simulink model "Octacopter"  (R2022b)
settings: Solver=VariableStepAuto  StartTime=0.0  StopTime=sim_time  RelTol=1e-3
values from neighbouring files (symbols this model uses):
  b = 1.2953*1e-5    (= 1.2953e-05)    [Junesh_Octacopter.m]    (also in Junesh_Octacopter.mat)
  d = 0.008    [Junesh_Octacopter.m]    (also in Junesh_Octacopter.mat)
  g = 9.81    [Junesh_Octacopter.m]    (also in Junesh_Octacopter.mat)
  Ixx = 0.0820    (= 0.082)    [Junesh_Octacopter.m]    (also in Junesh_Octacopter.mat)
  Iyy = 0.0845    [Junesh_Octacopter.m]    (also in Junesh_Octacopter.mat)
  Izz = 0.1377    [Junesh_Octacopter.m]    (also in Junesh_Octacopter.mat)
  Kdx = 0.50    (= 0.5)    [Junesh_Octacopter.m]    (also in Junesh_Octacopter.mat = 0.245)
  Kdy = 0.15    [Junesh_Octacopter.m]    (also in Junesh_Octacopter.mat = 0.8)
  Kip = 2    [Junesh_Octacopter.m]    (also in Junesh_Octacopter.mat = 20)
  Kiq = 2    [Junesh_Octacopter.m]    (also in Junesh_Octacopter.mat = 21)
  Kir = 2.2    [Junesh_Octacopter.m]    (also in Junesh_Octacopter.mat = 10.1)
  Kiz = 15    [Junesh_Octacopter.m]    (also in Junesh_Octacopter.mat = 500)
  Kop = 5    [Junesh_Octacopter.m]    (also in Junesh_Octacopter.mat = 39)
  Kopi = 0    [Junesh_Octacopter.m]    (also in Junesh_Octacopter.mat)
  Koq = 5    [Junesh_Octacopter.m]    (also in Junesh_Octacopter.mat = 38)
  Koqi = 0    [Junesh_Octacopter.m]    (also in Junesh_Octacopter.mat)
  Kor = 1    [Junesh_Octacopter.m]    (also in Junesh_Octacopter.mat = 3.6)
  Kori = 0    [Junesh_Octacopter.m]    (also in Junesh_Octacopter.mat)
  Koz = 1    [Junesh_Octacopter.m]    (also in Junesh_Octacopter.mat = 1.5)
  Kozi = 0    [Junesh_Octacopter.m]    (also in Junesh_Octacopter.mat)
  Kpx = 0.3    [Junesh_Octacopter.m]    (also in Junesh_Octacopter.mat = 0.061)
  Kpy = 0    [Junesh_Octacopter.m]    (also in Junesh_Octacopter.mat = 0.1)
  l = 0.315    [Junesh_Octacopter.m]    (also in Junesh_Octacopter.mat)
  m = 4.34    [Junesh_Octacopter.m]    (also in Junesh_Octacopter.mat)
settings Model: Creator=junes  LastModifiedBy=junes

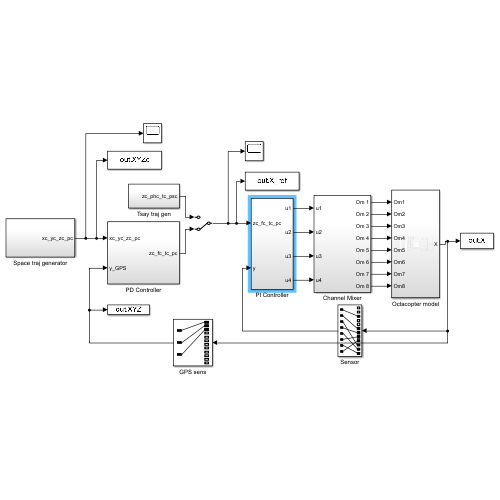
[thumbnail: Simulink's stored preview of the top-level diagram]
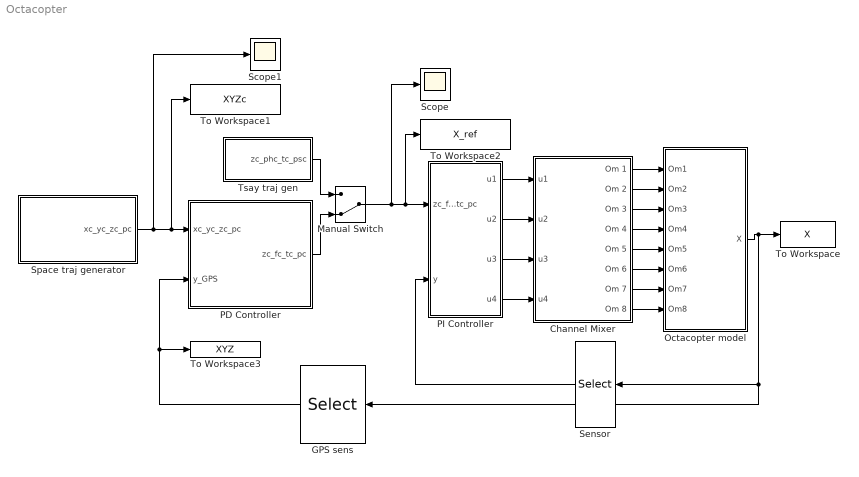
== system Octacopter ==
  Channel Mixer : Subsystem
  GPS sens : Selector  InputPortWidth=12  IndexOptions=Index vector (dialog)  Indices=[1 2 3]  OutputSizes=1
  Manual Switch : ManualSwitch  CurrentSetting=0
  Octacopter model : Subsystem
  PD Controller : Subsystem
  PI Controller : Subsystem
  Scope : Scope
  Scope1 : Scope
  Sensor : Selector  InputPortWidth=12  IndexOptions=Index vector (dialog)  Indices=[3 6 10 7 11 8 12 9]  OutputSizes=1
  Space traj generator : Subsystem
  To Workspace : ToWorkspace  VariableName=X  SampleTime=-1
  To Workspace1 : ToWorkspace  VariableName=XYZc  SampleTime=-1
  To Workspace2 : ToWorkspace  VariableName=X_ref  SampleTime=-1
  To Workspace3 : ToWorkspace  VariableName=XYZ  SampleTime=-1
  Tsay traj gen : Subsystem
  wires:
  Octacopter model/1(X) -> GPS sens/1, Sensor/1, To Workspace/1
  Space traj generator/1(xc_yc_zc_pc) -> To Workspace1/1, PD Controller/1(xc_yc_zc_pc), Scope1/1
  Tsay traj gen/1(zc_phc_tc_psc) -> Manual Switch/1
  GPS sens/1 -> To Workspace3/1, PD Controller/2(y_GPS)
  Manual Switch/1 -> To Workspace2/1, PI Controller/1(zc_fc_tc_pc), Scope/1
  PD Controller/1(zc_fc_tc_pc) -> Manual Switch/2
  Sensor/1 -> PI Controller/2(y)
  Channel Mixer/1(Om 1) -> Octacopter model/1(Om1)
  Channel Mixer/2(Om 2) -> Octacopter model/2(Om2)
  Channel Mixer/3(Om 3) -> Octacopter model/3(Om3)
  Channel Mixer/4(Om 4) -> Octacopter model/4(Om4)
  Channel Mixer/5(Om 5) -> Octacopter model/5(Om5)
  Channel Mixer/6(Om 6) -> Octacopter model/6(Om6)
  Channel Mixer/7(Om 7) -> Octacopter model/7(Om7)
  Channel Mixer/8(Om 8) -> Octacopter model/8(Om8)
  PI Controller/2(u2) -> Channel Mixer/2(u2)
  PI Controller/1(u1) -> Channel Mixer/1(u1)
  PI Controller/3(u3) -> Channel Mixer/3(u3)
  PI Controller/4(u4) -> Channel Mixer/4(u4)

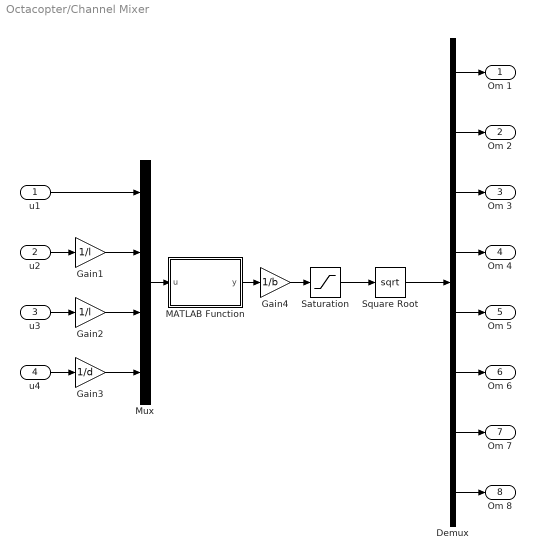
== system Octacopter/Channel Mixer ==
  u1 : Inport
  u2 : Inport  Port=2
  u3 : Inport  Port=3
  u4 : Inport  Port=4
  Demux : Demux  Outputs=8
  Gain1 : Gain  Gain=1/l
  Gain2 : Gain  Gain=1/l
  Gain3 : Gain  Gain=1/d
  Gain4 : Gain  Gain=1/b
  MATLAB Function : MATLAB Function  TreatAsAtomicUnit=on
  Mux : Mux
  Saturation : Saturate  UpperLimit=inf  LowerLimit=0
  Square Root : Sqrt
  Om 1 : Outport
  Om 2 : Outport  Port=2
  Om 3 : Outport  Port=3
  Om 4 : Outport  Port=4
  Om 5 : Outport  Port=5
  Om 6 : Outport  Port=6
  Om 7 : Outport  Port=7
  Om 8 : Outport  Port=8
  wires:
  Demux/8 -> Om 8/1
  Demux/7 -> Om 7/1
  Demux/1 -> Om 1/1
  Demux/2 -> Om 2/1
  Demux/5 -> Om 5/1
  Demux/4 -> Om 4/1
  Demux/6 -> Om 6/1
  MATLAB Function/1(y) -> Gain4/1
  Gain2/1 -> Mux/3
  u4/1 -> Gain3/1
  Gain3/1 -> Mux/4
  u1/1 -> Mux/1
  Gain1/1 -> Mux/2
  Gain4/1 -> Saturation/1
  u2/1 -> Gain1/1
  Mux/1 -> MATLAB Function/1(u)
  Demux/3 -> Om 3/1
  Saturation/1 -> Square Root/1
  Square Root/1 -> Demux/1
  u3/1 -> Gain2/1

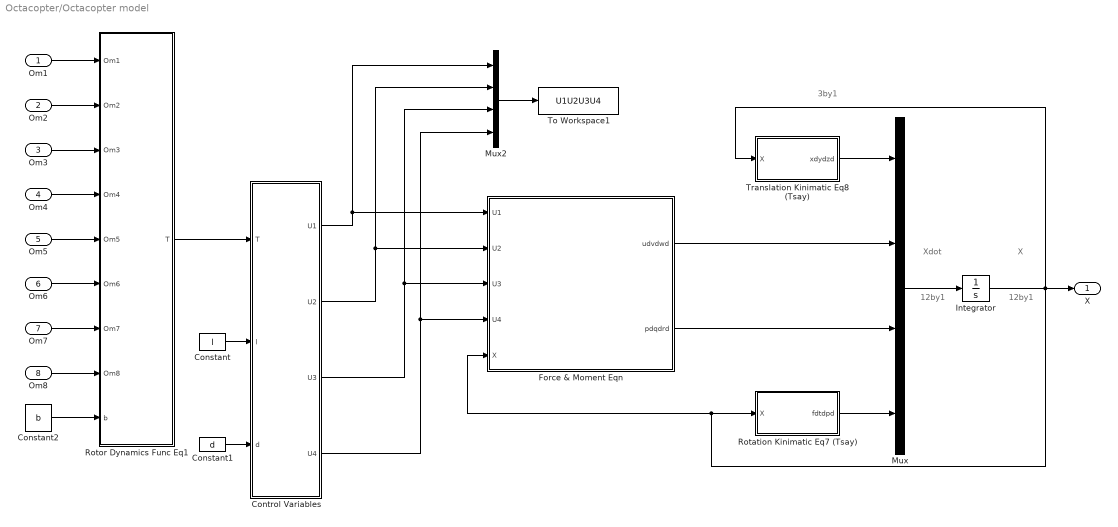
== system Octacopter/Octacopter model ==
  note: Xdot
  note: X
  note: 12by1
  note: 12by1
  note: 3by1
  Om1 : Inport
  Om2 : Inport  Port=2
  Om3 : Inport  Port=3
  Om4 : Inport  Port=4
  Om5 : Inport  Port=5
  Om6 : Inport  Port=6
  Om7 : Inport  Port=7
  Om8 : Inport  Port=8
  Constant : Constant  Value=l
  Constant1 : Constant  Value=d
  Constant2 : Constant  Value=b
  Control Variables : MATLAB Function  TreatAsAtomicUnit=on
  Force & Moment Eqn : Subsystem
  Integrator : Integrator  InitialCondition=zeros(12,1)
  Mux : Mux
  Mux2 : Mux
  Rotation Kinimatic Eq7 (Tsay) : MATLAB Function  TreatAsAtomicUnit=on
  Rotor Dynamics Func Eq1 : MATLAB Function  TreatAsAtomicUnit=on
  To Workspace1 : ToWorkspace  VariableName=U1U2U3U4  SampleTime=-1
  Translation Kinimatic Eq8 (Tsay) : MATLAB Function  TreatAsAtomicUnit=on
  X : Outport
  wires:
  Control Variables/2(U2) -> Mux2/2, Force & Moment Eqn/2(U2)
  Om1/1 -> Rotor Dynamics Func Eq1/1(Om1)
  Integrator/1 -> X/1, Force & Moment Eqn/5(X), Rotation Kinimatic Eq7 (Tsay)/1(X), Translation Kinimatic Eq8 (Tsay)/1(X)
  Rotor Dynamics Func Eq1/1(T) -> Control Variables/1(T)
  Force & Moment Eqn/1(udvdwd) -> Mux/2
  Force & Moment Eqn/2(pdqdrd) -> Mux/3
  Constant2/1 -> Rotor Dynamics Func Eq1/9(b)
  Mux2/1 -> To Workspace1/1
  Control Variables/1(U1) -> Mux2/1, Force & Moment Eqn/1(U1)
  Constant1/1 -> Control Variables/3(d)
  Constant/1 -> Control Variables/2(l)
  Rotation Kinimatic Eq7 (Tsay)/1(fdtdpd) -> Mux/4
  Control Variables/3(U3) -> Mux2/3, Force & Moment Eqn/3(U3)
  Om2/1 -> Rotor Dynamics Func Eq1/2(Om2)
  Mux/1 -> Integrator/1
  Translation Kinimatic Eq8 (Tsay)/1(xdydzd) -> Mux/1
  Control Variables/4(U4) -> Mux2/4, Force & Moment Eqn/4(U4)
  Om4/1 -> Rotor Dynamics Func Eq1/4(Om4)
  Om3/1 -> Rotor Dynamics Func Eq1/3(Om3)
  Om5/1 -> Rotor Dynamics Func Eq1/5(Om5)
  Om6/1 -> Rotor Dynamics Func Eq1/6(Om6)
  Om7/1 -> Rotor Dynamics Func Eq1/7(Om7)
  Om8/1 -> Rotor Dynamics Func Eq1/8(Om8)

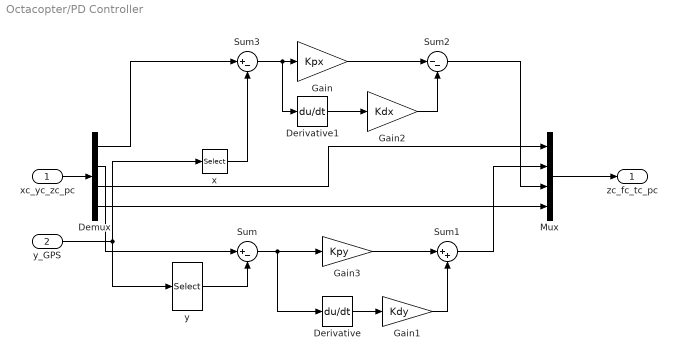
== system Octacopter/PD Controller ==
  xc_yc_zc_pc : Inport
  y_GPS : Inport  Port=2
  Demux : Demux
  Derivative : Derivative
  Derivative1 : Derivative
  Gain : Gain  Gain=Kpx
  Gain1 : Gain  Gain=Kdy
  Gain2 : Gain  Gain=Kdx
  Gain3 : Gain  Gain=Kpy
  Mux : Mux
  Sum : Sum  Inputs=|+-
  Sum1 : Sum  Inputs=|++
  Sum2 : Sum  Inputs=|--
  Sum3 : Sum  Inputs=|+-
  x : Selector  InputPortWidth=3  IndexOptions=Index vector (dialog)  Indices=1  OutputSizes=1
  y : Selector  InputPortWidth=3  IndexOptions=Index vector (dialog)  Indices=2  OutputSizes=1
  zc_fc_tc_pc : Outport
  wires:
  Demux/2 -> Sum/1
  Mux/1 -> zc_fc_tc_pc/1
  xc_yc_zc_pc/1 -> Demux/1
  Demux/3 -> Mux/1
  Demux/4 -> Mux/4
  y_GPS/1 -> x/1, y/1
  y/1 -> Sum/2
  Sum/1 -> Derivative/1, Gain3/1
  Derivative/1 -> Gain1/1
  Gain3/1 -> Sum1/1
  Gain1/1 -> Sum1/2
  Sum1/1 -> Mux/2
  Gain/1 -> Sum2/1
  Derivative1/1 -> Gain2/1
  Gain2/1 -> Sum2/2
  Demux/1 -> Sum3/1
  Sum3/1 -> Derivative1/1, Gain/1
  x/1 -> Sum3/2
  Sum2/1 -> Mux/3

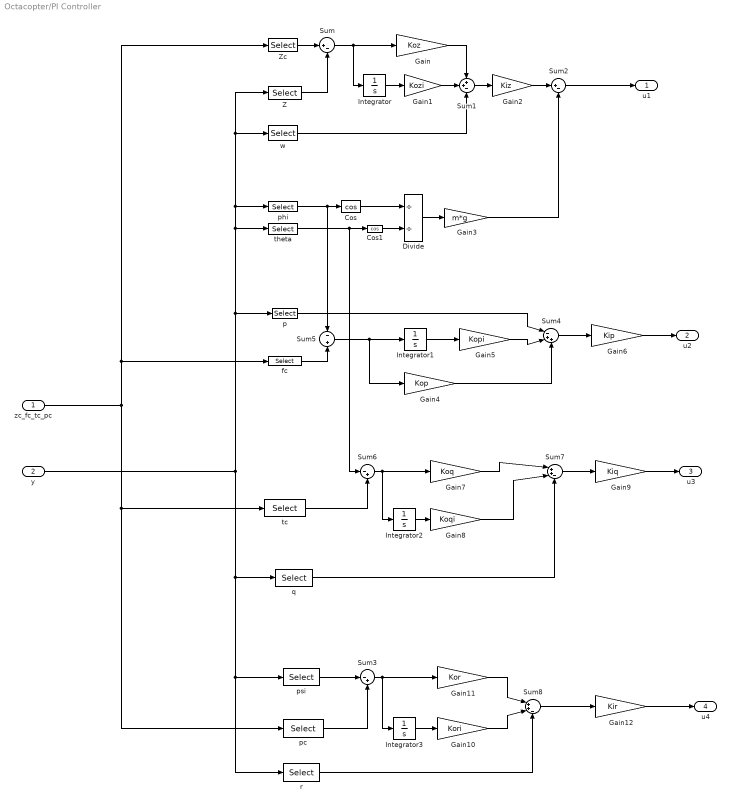
== system Octacopter/PI Controller ==
  zc_fc_tc_pc : Inport
  y : Inport  Port=2
  Cos : Trigonometry  Operator=cos
  Cos1 : Trigonometry  Operator=cos
  Divide : Product  Inputs=//
  Gain : Gain  Gain=Koz
  Gain1 : Gain  Gain=Kozi
  Gain10 : Gain  Gain=Kori
  Gain11 : Gain  Gain=Kor
  Gain12 : Gain  Gain=Kir
  Gain2 : Gain  Gain=Kiz
  Gain3 : Gain  Gain=m*g
  Gain4 : Gain  Gain=Kop
  Gain5 : Gain  Gain=Kopi
  Gain6 : Gain  Gain=Kip
  Gain7 : Gain  Gain=Koq
  Gain8 : Gain  Gain=Koqi
  Gain9 : Gain  Gain=Kiq
  Integrator{,1..3} (4 alike) : Integrator
  Sum : Sum  Inputs=|+-
  Sum1 : Sum  Inputs=++-
  Sum2 : Sum  Inputs=|+-
  Sum3 : Sum  Inputs=|-+
  Sum4 : Sum  Inputs=|-++
  Sum5 : Sum  Inputs=-+
  Sum6 : Sum  Inputs=|-+
  Sum7 : Sum  Inputs=|++-
  Sum8 : Sum  Inputs=|++-
  Z : Selector  InputPortWidth=8  IndexOptions=Index vector (dialog)  Indices=1  OutputSizes=1
  Zc : Selector  InputPortWidth=4  IndexOptions=Index vector (dialog)  Indices=1  OutputSizes=1
  fc : Selector  InputPortWidth=4  IndexOptions=Index vector (dialog)  Indices=2  OutputSizes=1
  p : Selector  InputPortWidth=8  IndexOptions=Index vector (dialog)  Indices=4  OutputSizes=1
  pc : Selector  InputPortWidth=4  IndexOptions=Index vector (dialog)  Indices=4  OutputSizes=1
  phi : Selector  InputPortWidth=8  IndexOptions=Index vector (dialog)  Indices=3  OutputSizes=1
  psi : Selector  InputPortWidth=8  IndexOptions=Index vector (dialog)  Indices=7  OutputSizes=1
  q : Selector  InputPortWidth=8  IndexOptions=Index vector (dialog)  Indices=6  OutputSizes=1
  r : Selector  InputPortWidth=8  IndexOptions=Index vector (dialog)  Indices=8  OutputSizes=1
  tc : Selector  InputPortWidth=4  IndexOptions=Index vector (dialog)  Indices=3  OutputSizes=1
  theta : Selector  InputPortWidth=8  IndexOptions=Index vector (dialog)  Indices=5  OutputSizes=1
  w : Selector  InputPortWidth=8  IndexOptions=Index vector (dialog)  Indices=2  OutputSizes=1
  u1 : Outport
  u2 : Outport  Port=2
  u3 : Outport  Port=3
  u4 : Outport  Port=4
  wires:
  Gain11/1 -> Sum8/1
  Integrator3/1 -> Gain10/1
  Gain12/1 -> u4/1
  fc/1 -> Sum5/2
  Gain10/1 -> Sum8/2
  Gain4/1 -> Sum4/3
  q/1 -> Sum7/3
  Sum6/1 -> Integrator2/1, Gain7/1
  Gain3/1 -> Sum2/2
  Integrator2/1 -> Gain8/1
  tc/1 -> Sum6/2
  Cos/1 -> Divide/1
  Divide/1 -> Gain3/1
  Gain7/1 -> Sum7/1
  Integrator1/1 -> Gain5/1
  Gain9/1 -> u3/1
  r/1 -> Sum8/3
  Gain6/1 -> u2/1
  Sum8/1 -> Gain12/1
  y/1 -> r/1, psi/1, q/1, Z/1, w/1, phi/1, theta/1, p/1
  phi/1 -> Cos/1, Sum5/1
  theta/1 -> Sum6/1, Cos1/1
  Sum/1 -> Integrator/1, Gain/1
  p/1 -> Sum4/1
  Sum3/1 -> Integrator3/1, Gain11/1
  Gain8/1 -> Sum7/2
  Gain/1 -> Sum1/1
  psi/1 -> Sum3/1
  Cos1/1 -> Divide/2
  Sum2/1 -> u1/1
  Sum1/1 -> Gain2/1
  w/1 -> Sum1/3
  Gain1/1 -> Sum1/2
  zc_fc_tc_pc/1 -> pc/1, tc/1, Zc/1, fc/1
  Sum5/1 -> Gain4/1, Integrator1/1
  Sum4/1 -> Gain6/1
  Gain5/1 -> Sum4/2
  Integrator/1 -> Gain1/1
  pc/1 -> Sum3/2
  Gain2/1 -> Sum2/1
  Z/1 -> Sum/2
  Sum7/1 -> Gain9/1
  Zc/1 -> Sum/1

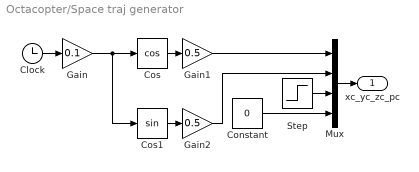
== system Octacopter/Space traj generator ==
  Clock : Clock
  Constant : Constant  Value=0
  Cos : Trigonometry  Operator=cos
  Cos1 : Trigonometry
  Gain : Gain  Gain=0.1
  Gain1 : Gain  Gain=0.5
  Gain2 : Gain  Gain=0.5
  Mux : Mux
  Step : Step  After=-9  SampleTime=0
  xc_yc_zc_pc : Outport
  wires:
  Mux/1 -> xc_yc_zc_pc/1
  Clock/1 -> Gain/1
  Gain/1 -> Cos1/1, Cos/1
  Cos/1 -> Gain1/1
  Gain1/1 -> Mux/1
  Cos1/1 -> Gain2/1
  Gain2/1 -> Mux/2
  Step/1 -> Mux/3
  Constant/1 -> Mux/4

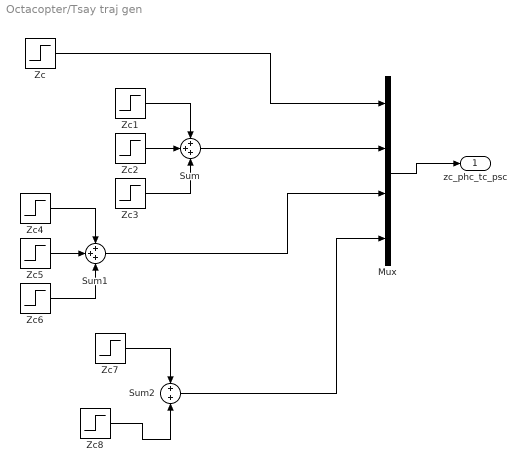
== system Octacopter/Tsay traj gen ==
  Mux : Mux
  Sum : Sum  Inputs=+++
  Sum1 : Sum  Inputs=+++
  Sum2 : Sum
  Zc : Step  After=-9  SampleTime=0
  Zc1 : Step  Time=20  After=5*pi/180  SampleTime=0
  Zc2 : Step  Time=40  After=-2*5*pi/180  SampleTime=0
  Zc3 : Step  Time=60  After=5*pi/180  SampleTime=0
  Zc4 : Step  Time=80  After=5*pi/180  SampleTime=0
  Zc5 : Step  Time=100  After=-2*5*pi/180  SampleTime=0
  Zc6 : Step  Time=120  After=5*pi/180  SampleTime=0
  Zc7 : Step  Time=150  After=45*pi/180  SampleTime=0
  Zc8 : Step  Time=170  After=-45*pi/180  SampleTime=0
  zc_phc_tc_psc : Outport
  wires:
  Mux/1 -> zc_phc_tc_psc/1
  Zc/1 -> Mux/1
  Zc1/1 -> Sum/1
  Zc2/1 -> Sum/2
  Zc3/1 -> Sum/3
  Sum/1 -> Mux/2
  Zc4/1 -> Sum1/1
  Sum1/1 -> Mux/3
  Zc6/1 -> Sum1/3
  Zc5/1 -> Sum1/2
  Zc7/1 -> Sum2/1
  Sum2/1 -> Mux/4
  Zc8/1 -> Sum2/2

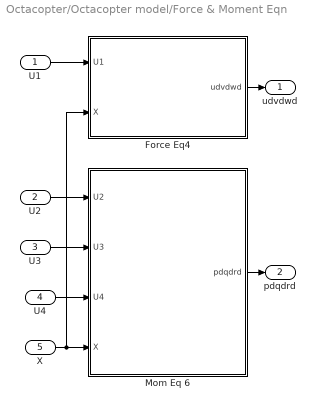
== system Octacopter/Octacopter model/Force & Moment Eqn ==
  U1 : Inport
  U2 : Inport  Port=2
  U3 : Inport  Port=3
  U4 : Inport  Port=4
  X : Inport  Port=5
  Force Eq4 : Subsystem
  Mom Eq 6 : Subsystem
  udvdwd : Outport
  pdqdrd : Outport  Port=2
  wires:
  Force Eq4/1(udvdwd) -> udvdwd/1
  Mom Eq 6/1(pdqdrd) -> pdqdrd/1
  U1/1 -> Force Eq4/1(U1)
  U2/1 -> Mom Eq 6/1(U2)
  U3/1 -> Mom Eq 6/2(U3)
  U4/1 -> Mom Eq 6/3(U4)
  X/1 -> Mom Eq 6/4(X), Force Eq4/2(X)

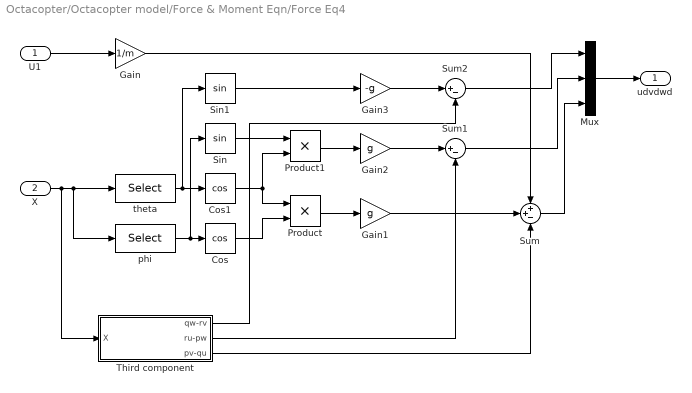
== system Octacopter/Octacopter model/Force & Moment Eqn/Force Eq4 ==
  U1 : Inport
  X : Inport  Port=2
  Cos : Trigonometry  Operator=cos
  Cos1 : Trigonometry  Operator=cos
  Gain : Gain  Gain=1/m
  Gain1 : Gain  Gain=g
  Gain2 : Gain  Gain=g
  Gain3 : Gain  Gain=-g
  Mux : Mux  Inputs=3
  Product : Product
  Product1 : Product
  Sin : Trigonometry
  Sin1 : Trigonometry
  Sum : Sum  Inputs=++-
  Sum1 : Sum  Inputs=|+-
  Sum2 : Sum  Inputs=|+-
  Third component : Subsystem
  phi : Selector  InputPortWidth=12  IndexOptions=Index vector (dialog)  Indices=10  OutputSizes=1
  theta : Selector  InputPortWidth=12  IndexOptions=Index vector (dialog)  Indices=11  OutputSizes=1
  udvdwd : Outport
  wires:
  Cos/1 -> Product/2
  theta/1 -> Cos1/1, Sin1/1
  Cos1/1 -> Product1/2, Product/1
  U1/1 -> Gain/1
  phi/1 -> Sin/1, Cos/1
  X/1 -> Third component/1(X), phi/1, theta/1
  Third component/1(qw-rv) -> Sum2/2
  Sum2/1 -> Mux/1
  Gain/1 -> Sum/1
  Sin/1 -> Product1/1
  Sum1/1 -> Mux/2
  Sin1/1 -> Gain3/1
  Product1/1 -> Gain2/1
  Gain3/1 -> Sum2/1
  Third component/2(ru-pw) -> Sum1/2
  Sum/1 -> Mux/3
  Mux/1 -> udvdwd/1
  Gain2/1 -> Sum1/1
  Gain1/1 -> Sum/2
  Product/1 -> Gain1/1
  Third component/3(pv-qu) -> Sum/3

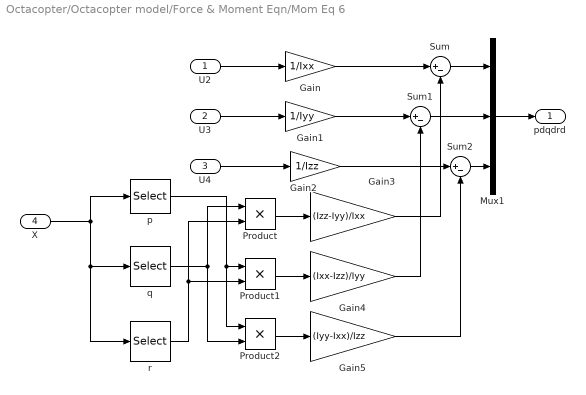
== system Octacopter/Octacopter model/Force & Moment Eqn/Mom Eq 6 ==
  U2 : Inport
  U3 : Inport  Port=2
  U4 : Inport  Port=3
  X : Inport  Port=4
  Gain : Gain  Gain=1/Ixx
  Gain1 : Gain  Gain=1/Iyy
  Gain2 : Gain  Gain=1/Izz
  Gain3 : Gain  Gain=(Izz-Iyy)/Ixx
  Gain4 : Gain  Gain=(Ixx-Izz)/Iyy
  Gain5 : Gain  Gain=(Iyy-Ixx)/Izz
  Mux1 : Mux  Inputs=3
  Product : Product
  Product1 : Product
  Product2 : Product
  Sum : Sum  Inputs=|+-
  Sum1 : Sum  Inputs=|+-
  Sum2 : Sum  Inputs=|+-
  p : Selector  InputPortWidth=12  IndexOptions=Index vector (dialog)  Indices=7  OutputSizes=1
  q : Selector  InputPortWidth=12  IndexOptions=Index vector (dialog)  Indices=8  OutputSizes=1
  r : Selector  InputPortWidth=12  IndexOptions=Index vector (dialog)  Indices=9  OutputSizes=1
  pdqdrd : Outport
  wires:
  Mux1/1 -> pdqdrd/1
  U2/1 -> Gain/1
  U3/1 -> Gain1/1
  U4/1 -> Gain2/1
  X/1 -> r/1, q/1, p/1
  Product/1 -> Gain3/1
  Gain/1 -> Sum/1
  Gain3/1 -> Sum/2
  Sum/1 -> Mux1/1
  Sum2/1 -> Mux1/3
  Sum1/1 -> Mux1/2
  Gain1/1 -> Sum1/1
  Gain2/1 -> Sum2/1
  Product1/1 -> Gain4/1
  Gain4/1 -> Sum1/2
  Gain5/1 -> Sum2/2
  Product2/1 -> Gain5/1
  q/1 -> Product2/2, Product/1
  r/1 -> Product1/2, Product/2
  p/1 -> Product2/1, Product1/1

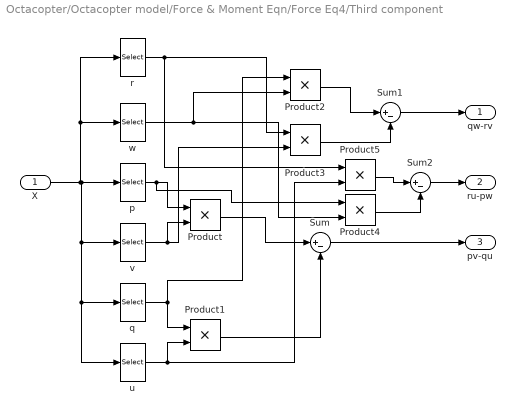
== system Octacopter/Octacopter model/Force & Moment Eqn/Force Eq4/Third component ==
  X : Inport
  Product{,1..5} (6 alike) : Product
  Sum : Sum  Inputs=|+-
  Sum1 : Sum  Inputs=|+-
  Sum2 : Sum  Inputs=|+-
  p : Selector  InputPortWidth=12  IndexOptions=Index vector (dialog)  Indices=7  OutputSizes=1
  q : Selector  InputPortWidth=12  IndexOptions=Index vector (dialog)  Indices=8  OutputSizes=1
  r : Selector  InputPortWidth=12  IndexOptions=Index vector (dialog)  Indices=9  OutputSizes=1
  u : Selector  InputPortWidth=12  IndexOptions=Index vector (dialog)  Indices=4  OutputSizes=1
  v : Selector  InputPortWidth=12  IndexOptions=Index vector (dialog)  Indices=5  OutputSizes=1
  w : Selector  InputPortWidth=12  IndexOptions=Index vector (dialog)  Indices=6  OutputSizes=1
  qw-rv : Outport
  ru-pw : Outport  Port=2
  pv-qu : Outport  Port=3
  wires:
  X/1 -> r/1, w/1, u/1, q/1, v/1, p/1
  p/1 -> Product4/1, Product/1
  v/1 -> Product3/2, Product/2
  u/1 -> Product5/2, Product1/2
  q/1 -> Product2/1, Product1/1
  Product/1 -> Sum/1
  Product1/1 -> Sum/2
  Sum/1 -> pv-qu/1
  w/1 -> Product4/2, Product2/2
  r/1 -> Product5/1, Product3/1
  Product2/1 -> Sum1/1
  Product3/1 -> Sum1/2
  Sum1/1 -> qw-rv/1
  Product4/1 -> Sum2/2
  Product5/1 -> Sum2/1
  Sum2/1 -> ru-pw/1

== matlab function Octacopter/Channel Mixer/MATLAB Function ==
  data: u input; y output
function y = fcn(u)
%#codegen
% A = [-1 -1 -1 -1 -1 -1 -1 -1;...
%      -1 -1  0  0  1  1  0  0;...
%       0  0 -1 -1  0  0  1  1;...
%      -1 -1  1  1 -1 -1  1  1];
A = [-0.1250   -0.2500         0   -0.1250;...
     -0.1250   -0.2500         0   -0.1250;...
     -0.1250    0.0000   -0.2500    0.1250;...
     -0.1250    0.0000   -0.2500    0.1250;...
     -0.1250    0.2500         0   -0.1250;...
     -0.1250    0.2500         0   -0.1250;...
     -0.1250    0.0000    0.2500    0.1250;...
     -0.1250    0.0000    0.2500    0.1250];

% A_inv = pinv(A);
% y = A_inv*u;

y = A*u;

== matlab function Octacopter/Octacopter model/Control Variables ==
  data: T input; U1 output; U2 output; U3 output; U4 output; l input; d input
function [U1,U2,U3,U4] = fcn(T, l, d)

T1 = T(1);
T2 = T(2);
T3 = T(3);
T4 = T(4);
T5 = T(5);
T6 = T(6);
T7 = T(7);
T8 = T(8);

U1 = -( T1 + T2 + T3 + T4 + T5 + T6 + T7 + T8);
U2 = l/2*(T6+T5-T1-T2);
U3 = l/2*(T7+T8-T4-T3);
U4 = d*(-T1 - T2 + T3 + T4 -T5 -T6 +T7 + T8);

end

== matlab function Octacopter/Octacopter model/Rotation Kinimatic Eq7 (Tsay) ==
  data: X input; fdtdpd output
function fdtdpd = fcn(X)
phi = X(10); 
theta = X(11); 
psi = X(12); 
p = X(7);
q = X(8);
r = X(9);
A = [1     tan(theta)*sin(phi)      tan(theta)*cos(phi);...
     0          cos(phi)            -sin(phi);...
     0     sec(theta)*sin(phi)     sec(theta)*cos(phi)];
b = [p q r]';
fdtdpd = A*b;

== matlab function Octacopter/Octacopter model/Rotor Dynamics Func Eq1 ==
  data: Om1 input; T output; Om2 input; Om3 input; Om4 input; Om5 input; Om6 input; Om7 input; Om8 input; b input
function T = fcn(Om1, Om2, Om3, Om4, Om5, Om6, Om7, Om8,b)


Om=[Om1,Om2,Om3,Om4,Om5,Om6,Om7,Om8];
T=[0,0,0,0,0,0,0,0];

i = 1;
while i<=8
    T(i) = Om(i)^2*b;
    i = i+1;

% T1 = b*Om1^2;
% T2 = b*Om2^2;
% T3 = b*Om3^2;
% T4 = b*Om4^2;

end

== matlab function Octacopter/Octacopter model/Translation Kinimatic Eq8 (Tsay) ==
  data: X input; xdydzd output
function xdydzd = fcn(X)
f = X(10); 
t = X(11);
p = X(12); 
u = X(4);
v = X(5);
w = X(6);
A = [cos(t)*cos(p)    sin(f)*sin(t)*cos(p)-cos(f)*sin(p)    cos(f)*sin(t)*cos(p)+sin(f)*sin(p);...
     cos(t)*sin(p)    cos(f)*cos(p)+sin(f)*sin(t)*sin(p)    cos(f)*sin(t)*sin(p)-sin(f)*cos(p);...
     -sin(t)                  sin(f)*cos(t)                          cos(f)*cos(t)            ];
b = [u v w]';
xdydzd = A*b;
